simulink library "xps_library"  (R2018a)
settings: Solver=ode45  StartTime=0.0  StopTime=10.0  RelTol=1e-3
undefined symbols (not defined in the file or in its folder): ip_name, lib_path
libraries: xbsIndex_r4 x2548, casper_library_flow_control x68, simulink x52, $bdroot x22, casper_library_misc x9
(part 4 of 30)

== system xps_library/ADCs/adc_mkid_4x ==
  conv : Subsystem
      mask help:
      | Converts an (12-bit) unsigned number to 2's complement.
      | This block should eventually be able to handle arbitrary
      | width inputs.
  conv1 : Subsystem
      mask help:
      | Converts an (12-bit) unsigned number to 2's complement.
      | This block should eventually be able to handle arbitrary
      | width inputs.
  conv2 : Subsystem
      mask help:
      | Converts an (12-bit) unsigned number to 2's complement.
      | This block should eventually be able to handle arbitrary
      | width inputs.
  conv3 : Subsystem
      mask help:
      | Converts an (12-bit) unsigned number to 2's complement.
      | This block should eventually be able to handle arbitrary
      | width inputs.
  conv4 : Subsystem
      mask help:
      | Converts an (12-bit) unsigned number to 2's complement.
      | This block should eventually be able to handle arbitrary
      | width inputs.
  conv5 : Subsystem
      mask help:
      | Converts an (12-bit) unsigned number to 2's complement.
      | This block should eventually be able to handle arbitrary
      | width inputs.
  conv6 : Subsystem
      mask help:
      | Converts an (12-bit) unsigned number to 2's complement.
      | This block should eventually be able to handle arbitrary
      | width inputs.
  conv7 : Subsystem
      mask help:
      | Converts an (12-bit) unsigned number to 2's complement.
      | This block should eventually be able to handle arbitrary
      | width inputs.
  xps_library_ADCs_adc_mkid_4x_user_data_i{0..3} (4 alike) : xbsIndex_r4/Gateway In  gui_display_data_type=Fixed-point  arith_type=Unsigned  n_bits=12  bin_pt=0  preci_type=Single  exp_width=8  frac_width=24  rows=1  columns=1  quantization=Truncate  overflow=Wrap  period=1  UseAsADC=off  ADCChannel='1'  interface=None  automatic_assignment=on  address_offset=hex2dec('00')  intf_name=''  intf_description=''  default_value=0  timing_constraint=None  locs_specified=off  LOCs={}  io_standard={}  inherit_from_input=off  hdl_port=on  dbl_ovrd=off  block_type=gatewayin
      settings: infoedit="Gateway in block.  Converts inputs of type Simulink integer, double and fixed point to  Xilinx fixed point type.<P><P>Hardware notes:  In hardware these blocks become top level input ports."  xl_area=[0, 0, 0, 0, 0, 0, 0]  block_version=10.1.3
  xps_library_ADCs_adc_mkid_4x_user_data_q{0..3} (4 alike) : xbsIndex_r4/Gateway In  gui_display_data_type=Fixed-point  arith_type=Unsigned  n_bits=12  bin_pt=0  preci_type=Single  exp_width=8  frac_width=24  rows=1  columns=1  quantization=Truncate  overflow=Wrap  period=1  UseAsADC=off  ADCChannel='1'  interface=None  automatic_assignment=on  address_offset=hex2dec('00')  intf_name=''  intf_description=''  default_value=0  timing_constraint=None  locs_specified=off  LOCs={}  io_standard={}  inherit_from_input=off  hdl_port=on  dbl_ovrd=off  block_type=gatewayin
      settings: infoedit="Gateway in block.  Converts inputs of type Simulink integer, double and fixed point to  Xilinx fixed point type.<P><P>Hardware notes:  In hardware these blocks become top level input ports."  xl_area=[0, 0, 0, 0, 0, 0, 0]  block_version=10.1.3
  xps_library_ADCs_adc_mkid_4x_user_sync : xbsIndex_r4/Gateway In  gui_display_data_type=Fixed-point  arith_type=Boolean  n_bits=1  bin_pt=0  preci_type=Single  exp_width=8  frac_width=24  rows=1  columns=1  quantization=Truncate  overflow=Wrap  period=1  UseAsADC=off  ADCChannel='1'  interface=None  automatic_assignment=on  address_offset=hex2dec('00')  intf_name=''  intf_description=''  default_value=0  timing_constraint=None  locs_specified=off  LOCs={}  io_standard={}  inherit_from_input=off  hdl_port=on  dbl_ovrd=off  block_type=gatewayin
      settings: infoedit="Gateway in block.  Converts inputs of type Simulink integer, double and fixed point to  Xilinx fixed point type.<P><P>Hardware notes:  In hardware these blocks become top level input ports."  xl_area=[0, 0, 0, 0, 0, 0, 0]  block_version=10.1.3
  data_i0 : Outport
  data_i1 : Outport  Port=2
  data_i2 : Outport  Port=3
  data_i3 : Outport  Port=4
  data_q0 : Outport  Port=5
  data_q1 : Outport  Port=6
  data_q2 : Outport  Port=7
  data_q3 : Outport  Port=8
  sync : Outport  Port=9
  wires:
  xps_library_ADCs_adc_mkid_4x_user_data_q3/1 -> conv7/1(In1)
  conv7/1(Out1) -> data_q3/1
  xps_library_ADCs_adc_mkid_4x_user_data_q2/1 -> conv6/1(In1)
  conv6/1(Out1) -> data_q2/1
  xps_library_ADCs_adc_mkid_4x_user_data_i3/1 -> conv5/1(In1)
  conv5/1(Out1) -> data_i3/1
  xps_library_ADCs_adc_mkid_4x_user_data_i2/1 -> conv4/1(In1)
  conv4/1(Out1) -> data_i2/1
  xps_library_ADCs_adc_mkid_4x_user_sync/1 -> sync/1
  xps_library_ADCs_adc_mkid_4x_user_data_i0/1 -> conv/1(In1)
  conv/1(Out1) -> data_i0/1
  xps_library_ADCs_adc_mkid_4x_user_data_q0/1 -> conv2/1(In1)
  conv2/1(Out1) -> data_q0/1
  xps_library_ADCs_adc_mkid_4x_user_data_i1/1 -> conv1/1(In1)
  conv1/1(Out1) -> data_i1/1
  xps_library_ADCs_adc_mkid_4x_user_data_q1/1 -> conv3/1(In1)
  conv3/1(Out1) -> data_q1/1

== system xps_library/ADCs/adc_sim ==
  sim_adc_data_in : Inport
  adc_bias : Bias  Bias=128  SaturateOnIntegerOverflow=on
  adc_gain : Gain  Gain=128
  overflow_detector : $bdroot/ADCs/of_detect_bus  nStreams=8  bit_width=8
  sample0_ds : DownSample  N=8  phase=1
  sample1_ds : DownSample  N=8  phase=2
  sample2_ds : DownSample  N=8  phase=3
  sample3_ds : DownSample  N=8  phase=4
  sample4_ds : DownSample  N=8  phase=5
  sample5_ds : DownSample  N=8  phase=6
  sample6_ds : DownSample  N=8  phase=7
  sample7_ds : DownSample  N=8
  s0 : Outport
  s1 : Outport  Port=2
  s2 : Outport  Port=3
  s3 : Outport  Port=4
  s4 : Outport  Port=5
  s5 : Outport  Port=6
  s6 : Outport  Port=7
  s7 : Outport  Port=8
  of : Outport  Port=9
  wires:
  sim_adc_data_in/1 -> adc_gain/1
  adc_gain/1 -> adc_bias/1
  overflow_detector/1 -> of/1
  adc_bias/1 -> sample0_ds/1, sample1_ds/1, sample2_ds/1, sample3_ds/1, sample4_ds/1, sample5_ds/1, sample6_ds/1, sample7_ds/1
  sample0_ds/1 -> overflow_detector/1, s0/1
  sample1_ds/1 -> overflow_detector/2, s1/1
  sample2_ds/1 -> overflow_detector/3, s2/1
  sample3_ds/1 -> overflow_detector/4, s3/1
  sample4_ds/1 -> overflow_detector/5, s4/1
  sample5_ds/1 -> overflow_detector/6, s5/1
  sample6_ds/1 -> overflow_detector/7, s6/1
  sample7_ds/1 -> overflow_detector/8, s7/1

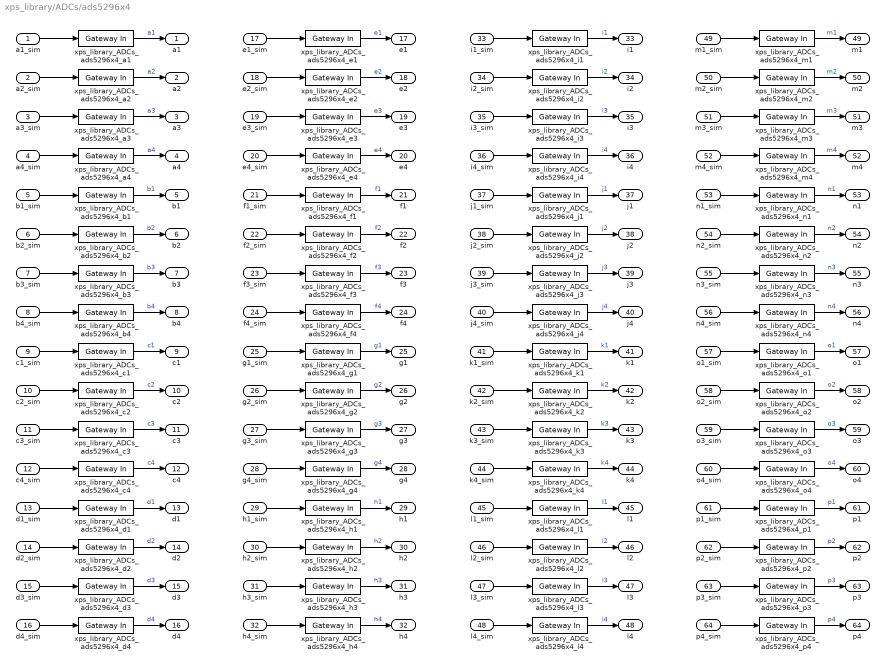
== system xps_library/ADCs/ads5296x4 ==
  a1_sim : Inport
  a2_sim : Inport  Port=2
  a3_sim : Inport  Port=3
  a4_sim : Inport  Port=4
  b1_sim : Inport  Port=5
  b2_sim : Inport  Port=6
  b3_sim : Inport  Port=7
  b4_sim : Inport  Port=8
  c1_sim : Inport  Port=9
  c2_sim : Inport  Port=10
  c3_sim : Inport  Port=11
  c4_sim : Inport  Port=12
  d1_sim : Inport  Port=13
  d2_sim : Inport  Port=14
  d3_sim : Inport  Port=15
  d4_sim : Inport  Port=16
  e1_sim : Inport  Port=17
  e2_sim : Inport  Port=18
  e3_sim : Inport  Port=19
  e4_sim : Inport  Port=20
  f1_sim : Inport  Port=21
  f2_sim : Inport  Port=22
  f3_sim : Inport  Port=23
  f4_sim : Inport  Port=24
  g1_sim : Inport  Port=25
  g2_sim : Inport  Port=26
  g3_sim : Inport  Port=27
  g4_sim : Inport  Port=28
  h1_sim : Inport  Port=29
  h2_sim : Inport  Port=30
  h3_sim : Inport  Port=31
  h4_sim : Inport  Port=32
  i1_sim : Inport  Port=33
  i2_sim : Inport  Port=34
  i3_sim : Inport  Port=35
  i4_sim : Inport  Port=36
  j1_sim : Inport  Port=37
  j2_sim : Inport  Port=38
  j3_sim : Inport  Port=39
  j4_sim : Inport  Port=40
  k1_sim : Inport  Port=41
  k2_sim : Inport  Port=42
  k3_sim : Inport  Port=43
  k4_sim : Inport  Port=44
  l1_sim : Inport  Port=45
  l2_sim : Inport  Port=46
  l3_sim : Inport  Port=47
  l4_sim : Inport  Port=48
  m1_sim : Inport  Port=49
  m2_sim : Inport  Port=50
  m3_sim : Inport  Port=51
  m4_sim : Inport  Port=52
  n1_sim : Inport  Port=53
  n2_sim : Inport  Port=54
  n3_sim : Inport  Port=55
  n4_sim : Inport  Port=56
  o1_sim : Inport  Port=57
  o2_sim : Inport  Port=58
  o3_sim : Inport  Port=59
  o4_sim : Inport  Port=60
  p1_sim : Inport  Port=61
  p2_sim : Inport  Port=62
  p3_sim : Inport  Port=63
  p4_sim : Inport  Port=64
  xps_library_ADCs_ads5296x4_a{1..4} (4 alike) : xbsIndex_r4/Gateway In  gui_display_data_type=Fixed-point  arith_type="Signed  (2's comp)"  n_bits=10  bin_pt=9  preci_type=Single  exp_width=8  frac_width=24  rows=1  columns=1  quantization="Round  (unbiased: +/- Inf)"  overflow=Saturate  period=1  UseAsADC=off  ADCChannel='1'  interface=None  automatic_assignment=on  address_offset=hex2dec('00')  intf_name=''  intf_description=''  default_value=0  timing_constraint=None  locs_specified=off  LOCs={}  io_standard={}  inherit_from_input=off  hdl_port=on  dbl_ovrd=off  block_type=gatewayin
  xps_library_ADCs_ads5296x4_b{1..4} (4 alike) : xbsIndex_r4/Gateway In  gui_display_data_type=Fixed-point  arith_type="Signed  (2's comp)"  n_bits=10  bin_pt=9  preci_type=Single  exp_width=8  frac_width=24  rows=1  columns=1  quantization="Round  (unbiased: +/- Inf)"  overflow=Saturate  period=1  UseAsADC=off  ADCChannel='1'  interface=None  automatic_assignment=on  address_offset=hex2dec('00')  intf_name=''  intf_description=''  default_value=0  timing_constraint=None  locs_specified=off  LOCs={}  io_standard={}  inherit_from_input=off  hdl_port=on  dbl_ovrd=off  block_type=gatewayin
  xps_library_ADCs_ads5296x4_c{1..4} (4 alike) : xbsIndex_r4/Gateway In  gui_display_data_type=Fixed-point  arith_type="Signed  (2's comp)"  n_bits=10  bin_pt=9  preci_type=Single  exp_width=8  frac_width=24  rows=1  columns=1  quantization="Round  (unbiased: +/- Inf)"  overflow=Saturate  period=1  UseAsADC=off  ADCChannel='1'  interface=None  automatic_assignment=on  address_offset=hex2dec('00')  intf_name=''  intf_description=''  default_value=0  timing_constraint=None  locs_specified=off  LOCs={}  io_standard={}  inherit_from_input=off  hdl_port=on  dbl_ovrd=off  block_type=gatewayin
  xps_library_ADCs_ads5296x4_d{1..4} (4 alike) : xbsIndex_r4/Gateway In  gui_display_data_type=Fixed-point  arith_type="Signed  (2's comp)"  n_bits=10  bin_pt=9  preci_type=Single  exp_width=8  frac_width=24  rows=1  columns=1  quantization="Round  (unbiased: +/- Inf)"  overflow=Saturate  period=1  UseAsADC=off  ADCChannel='1'  interface=None  automatic_assignment=on  address_offset=hex2dec('00')  intf_name=''  intf_description=''  default_value=0  timing_constraint=None  locs_specified=off  LOCs={}  io_standard={}  inherit_from_input=off  hdl_port=on  dbl_ovrd=off  block_type=gatewayin
  xps_library_ADCs_ads5296x4_e{1..4} (4 alike) : xbsIndex_r4/Gateway In  gui_display_data_type=Fixed-point  arith_type="Signed  (2's comp)"  n_bits=10  bin_pt=9  preci_type=Single  exp_width=8  frac_width=24  rows=1  columns=1  quantization="Round  (unbiased: +/- Inf)"  overflow=Saturate  period=1  UseAsADC=off  ADCChannel='1'  interface=None  automatic_assignment=on  address_offset=hex2dec('00')  intf_name=''  intf_description=''  default_value=0  timing_constraint=None  locs_specified=off  LOCs={}  io_standard={}  inherit_from_input=off  hdl_port=on  dbl_ovrd=off  block_type=gatewayin
  xps_library_ADCs_ads5296x4_f{1..4} (4 alike) : xbsIndex_r4/Gateway In  gui_display_data_type=Fixed-point  arith_type="Signed  (2's comp)"  n_bits=10  bin_pt=9  preci_type=Single  exp_width=8  frac_width=24  rows=1  columns=1  quantization="Round  (unbiased: +/- Inf)"  overflow=Saturate  period=1  UseAsADC=off  ADCChannel='1'  interface=None  automatic_assignment=on  address_offset=hex2dec('00')  intf_name=''  intf_description=''  default_value=0  timing_constraint=None  locs_specified=off  LOCs={}  io_standard={}  inherit_from_input=off  hdl_port=on  dbl_ovrd=off  block_type=gatewayin
  xps_library_ADCs_ads5296x4_g{1..4} (4 alike) : xbsIndex_r4/Gateway In  gui_display_data_type=Fixed-point  arith_type="Signed  (2's comp)"  n_bits=10  bin_pt=9  preci_type=Single  exp_width=8  frac_width=24  rows=1  columns=1  quantization="Round  (unbiased: +/- Inf)"  overflow=Saturate  period=1  UseAsADC=off  ADCChannel='1'  interface=None  automatic_assignment=on  address_offset=hex2dec('00')  intf_name=''  intf_description=''  default_value=0  timing_constraint=None  locs_specified=off  LOCs={}  io_standard={}  inherit_from_input=off  hdl_port=on  dbl_ovrd=off  block_type=gatewayin
  xps_library_ADCs_ads5296x4_h{1..4} (4 alike) : xbsIndex_r4/Gateway In  gui_display_data_type=Fixed-point  arith_type="Signed  (2's comp)"  n_bits=10  bin_pt=9  preci_type=Single  exp_width=8  frac_width=24  rows=1  columns=1  quantization="Round  (unbiased: +/- Inf)"  overflow=Saturate  period=1  UseAsADC=off  ADCChannel='1'  interface=None  automatic_assignment=on  address_offset=hex2dec('00')  intf_name=''  intf_description=''  default_value=0  timing_constraint=None  locs_specified=off  LOCs={}  io_standard={}  inherit_from_input=off  hdl_port=on  dbl_ovrd=off  block_type=gatewayin
  xps_library_ADCs_ads5296x4_i{1..4} (4 alike) : xbsIndex_r4/Gateway In  gui_display_data_type=Fixed-point  arith_type="Signed  (2's comp)"  n_bits=10  bin_pt=9  preci_type=Single  exp_width=8  frac_width=24  rows=1  columns=1  quantization="Round  (unbiased: +/- Inf)"  overflow=Saturate  period=1  UseAsADC=off  ADCChannel='1'  interface=None  automatic_assignment=on  address_offset=hex2dec('00')  intf_name=''  intf_description=''  default_value=0  timing_constraint=None  locs_specified=off  LOCs={}  io_standard={}  inherit_from_input=off  hdl_port=on  dbl_ovrd=off  block_type=gatewayin
  xps_library_ADCs_ads5296x4_j{1..4} (4 alike) : xbsIndex_r4/Gateway In  gui_display_data_type=Fixed-point  arith_type="Signed  (2's comp)"  n_bits=10  bin_pt=9  preci_type=Single  exp_width=8  frac_width=24  rows=1  columns=1  quantization="Round  (unbiased: +/- Inf)"  overflow=Saturate  period=1  UseAsADC=off  ADCChannel='1'  interface=None  automatic_assignment=on  address_offset=hex2dec('00')  intf_name=''  intf_description=''  default_value=0  timing_constraint=None  locs_specified=off  LOCs={}  io_standard={}  inherit_from_input=off  hdl_port=on  dbl_ovrd=off  block_type=gatewayin
  xps_library_ADCs_ads5296x4_k{1..4} (4 alike) : xbsIndex_r4/Gateway In  gui_display_data_type=Fixed-point  arith_type="Signed  (2's comp)"  n_bits=10  bin_pt=9  preci_type=Single  exp_width=8  frac_width=24  rows=1  columns=1  quantization="Round  (unbiased: +/- Inf)"  overflow=Saturate  period=1  UseAsADC=off  ADCChannel='1'  interface=None  automatic_assignment=on  address_offset=hex2dec('00')  intf_name=''  intf_description=''  default_value=0  timing_constraint=None  locs_specified=off  LOCs={}  io_standard={}  inherit_from_input=off  hdl_port=on  dbl_ovrd=off  block_type=gatewayin
  xps_library_ADCs_ads5296x4_l{1..4} (4 alike) : xbsIndex_r4/Gateway In  gui_display_data_type=Fixed-point  arith_type="Signed  (2's comp)"  n_bits=10  bin_pt=9  preci_type=Single  exp_width=8  frac_width=24  rows=1  columns=1  quantization="Round  (unbiased: +/- Inf)"  overflow=Saturate  period=1  UseAsADC=off  ADCChannel='1'  interface=None  automatic_assignment=on  address_offset=hex2dec('00')  intf_name=''  intf_description=''  default_value=0  timing_constraint=None  locs_specified=off  LOCs={}  io_standard={}  inherit_from_input=off  hdl_port=on  dbl_ovrd=off  block_type=gatewayin
  xps_library_ADCs_ads5296x4_m{1..4} (4 alike) : xbsIndex_r4/Gateway In  gui_display_data_type=Fixed-point  arith_type="Signed  (2's comp)"  n_bits=10  bin_pt=9  preci_type=Single  exp_width=8  frac_width=24  rows=1  columns=1  quantization="Round  (unbiased: +/- Inf)"  overflow=Saturate  period=1  UseAsADC=off  ADCChannel='1'  interface=None  automatic_assignment=on  address_offset=hex2dec('00')  intf_name=''  intf_description=''  default_value=0  timing_constraint=None  locs_specified=off  LOCs={}  io_standard={}  inherit_from_input=off  hdl_port=on  dbl_ovrd=off  block_type=gatewayin
  xps_library_ADCs_ads5296x4_n{1..4} (4 alike) : xbsIndex_r4/Gateway In  gui_display_data_type=Fixed-point  arith_type="Signed  (2's comp)"  n_bits=10  bin_pt=9  preci_type=Single  exp_width=8  frac_width=24  rows=1  columns=1  quantization="Round  (unbiased: +/- Inf)"  overflow=Saturate  period=1  UseAsADC=off  ADCChannel='1'  interface=None  automatic_assignment=on  address_offset=hex2dec('00')  intf_name=''  intf_description=''  default_value=0  timing_constraint=None  locs_specified=off  LOCs={}  io_standard={}  inherit_from_input=off  hdl_port=on  dbl_ovrd=off  block_type=gatewayin
  xps_library_ADCs_ads5296x4_o{1..4} (4 alike) : xbsIndex_r4/Gateway In  gui_display_data_type=Fixed-point  arith_type="Signed  (2's comp)"  n_bits=10  bin_pt=9  preci_type=Single  exp_width=8  frac_width=24  rows=1  columns=1  quantization="Round  (unbiased: +/- Inf)"  overflow=Saturate  period=1  UseAsADC=off  ADCChannel='1'  interface=None  automatic_assignment=on  address_offset=hex2dec('00')  intf_name=''  intf_description=''  default_value=0  timing_constraint=None  locs_specified=off  LOCs={}  io_standard={}  inherit_from_input=off  hdl_port=on  dbl_ovrd=off  block_type=gatewayin
  xps_library_ADCs_ads5296x4_p{1..4} (4 alike) : xbsIndex_r4/Gateway In  gui_display_data_type=Fixed-point  arith_type="Signed  (2's comp)"  n_bits=10  bin_pt=9  preci_type=Single  exp_width=8  frac_width=24  rows=1  columns=1  quantization="Round  (unbiased: +/- Inf)"  overflow=Saturate  period=1  UseAsADC=off  ADCChannel='1'  interface=None  automatic_assignment=on  address_offset=hex2dec('00')  intf_name=''  intf_description=''  default_value=0  timing_constraint=None  locs_specified=off  LOCs={}  io_standard={}  inherit_from_input=off  hdl_port=on  dbl_ovrd=off  block_type=gatewayin
  a1 : Outport
  a2 : Outport  Port=2
  a3 : Outport  Port=3
  a4 : Outport  Port=4
  b1 : Outport  Port=5
  b2 : Outport  Port=6
  b3 : Outport  Port=7
  b4 : Outport  Port=8
  c1 : Outport  Port=9
  c2 : Outport  Port=10
  c3 : Outport  Port=11
  c4 : Outport  Port=12
  d1 : Outport  Port=13
  d2 : Outport  Port=14
  d3 : Outport  Port=15
  d4 : Outport  Port=16
  e1 : Outport  Port=17
  e2 : Outport  Port=18
  e3 : Outport  Port=19
  e4 : Outport  Port=20
  f1 : Outport  Port=21
  f2 : Outport  Port=22
  f3 : Outport  Port=23
  f4 : Outport  Port=24
  g1 : Outport  Port=25
  g2 : Outport  Port=26
  g3 : Outport  Port=27
  g4 : Outport  Port=28
  h1 : Outport  Port=29
  h2 : Outport  Port=30
  h3 : Outport  Port=31
  h4 : Outport  Port=32
  i1 : Outport  Port=33
  i2 : Outport  Port=34
  i3 : Outport  Port=35
  i4 : Outport  Port=36
  j1 : Outport  Port=37
  j2 : Outport  Port=38
  j3 : Outport  Port=39
  j4 : Outport  Port=40
  k1 : Outport  Port=41
  k2 : Outport  Port=42
  k3 : Outport  Port=43
  k4 : Outport  Port=44
  l1 : Outport  Port=45
  l2 : Outport  Port=46
  l3 : Outport  Port=47
  l4 : Outport  Port=48
  m1 : Outport  Port=49
  m2 : Outport  Port=50
  m3 : Outport  Port=51
  m4 : Outport  Port=52
  n1 : Outport  Port=53
  n2 : Outport  Port=54
  n3 : Outport  Port=55
  n4 : Outport  Port=56
  o1 : Outport  Port=57
  o2 : Outport  Port=58
  o3 : Outport  Port=59
  o4 : Outport  Port=60
  p1 : Outport  Port=61
  p2 : Outport  Port=62
  p3 : Outport  Port=63
  p4 : Outport  Port=64
  wires:
  a1_sim/1 -> xps_library_ADCs_ads5296x4_a1/1
  xps_library_ADCs_ads5296x4_a1/1 -> a1/1  "a1"
  a2_sim/1 -> xps_library_ADCs_ads5296x4_a2/1
  xps_library_ADCs_ads5296x4_a2/1 -> a2/1  "a2"
  a3_sim/1 -> xps_library_ADCs_ads5296x4_a3/1
  xps_library_ADCs_ads5296x4_a3/1 -> a3/1  "a3"
  a4_sim/1 -> xps_library_ADCs_ads5296x4_a4/1
  xps_library_ADCs_ads5296x4_a4/1 -> a4/1  "a4"
  b1_sim/1 -> xps_library_ADCs_ads5296x4_b1/1
  xps_library_ADCs_ads5296x4_b1/1 -> b1/1  "b1"
  b2_sim/1 -> xps_library_ADCs_ads5296x4_b2/1
  xps_library_ADCs_ads5296x4_b2/1 -> b2/1  "b2"
  b3_sim/1 -> xps_library_ADCs_ads5296x4_b3/1
  xps_library_ADCs_ads5296x4_b3/1 -> b3/1  "b3"
  b4_sim/1 -> xps_library_ADCs_ads5296x4_b4/1
  xps_library_ADCs_ads5296x4_b4/1 -> b4/1  "b4"
  c1_sim/1 -> xps_library_ADCs_ads5296x4_c1/1
  xps_library_ADCs_ads5296x4_c1/1 -> c1/1  "c1"
  c2_sim/1 -> xps_library_ADCs_ads5296x4_c2/1
  xps_library_ADCs_ads5296x4_c2/1 -> c2/1  "c2"
  c3_sim/1 -> xps_library_ADCs_ads5296x4_c3/1
  xps_library_ADCs_ads5296x4_c3/1 -> c3/1  "c3"
  c4_sim/1 -> xps_library_ADCs_ads5296x4_c4/1
  xps_library_ADCs_ads5296x4_c4/1 -> c4/1  "c4"
  d1_sim/1 -> xps_library_ADCs_ads5296x4_d1/1
  xps_library_ADCs_ads5296x4_d1/1 -> d1/1  "d1"
  d2_sim/1 -> xps_library_ADCs_ads5296x4_d2/1
  xps_library_ADCs_ads5296x4_d2/1 -> d2/1  "d2"
  d3_sim/1 -> xps_library_ADCs_ads5296x4_d3/1
  xps_library_ADCs_ads5296x4_d3/1 -> d3/1  "d3"
  d4_sim/1 -> xps_library_ADCs_ads5296x4_d4/1
  xps_library_ADCs_ads5296x4_d4/1 -> d4/1  "d4"
  e1_sim/1 -> xps_library_ADCs_ads5296x4_e1/1
  xps_library_ADCs_ads5296x4_e1/1 -> e1/1  "e1"
  e2_sim/1 -> xps_library_ADCs_ads5296x4_e2/1
  xps_library_ADCs_ads5296x4_e2/1 -> e2/1  "e2"
  e3_sim/1 -> xps_library_ADCs_ads5296x4_e3/1
  xps_library_ADCs_ads5296x4_e3/1 -> e3/1  "e3"
  e4_sim/1 -> xps_library_ADCs_ads5296x4_e4/1
  xps_library_ADCs_ads5296x4_e4/1 -> e4/1  "e4"
  f1_sim/1 -> xps_library_ADCs_ads5296x4_f1/1
  xps_library_ADCs_ads5296x4_f1/1 -> f1/1  "f1"
  f2_sim/1 -> xps_library_ADCs_ads5296x4_f2/1
  xps_library_ADCs_ads5296x4_f2/1 -> f2/1  "f2"
  f3_sim/1 -> xps_library_ADCs_ads5296x4_f3/1
  xps_library_ADCs_ads5296x4_f3/1 -> f3/1  "f3"
  f4_sim/1 -> xps_library_ADCs_ads5296x4_f4/1
  xps_library_ADCs_ads5296x4_f4/1 -> f4/1  "f4"
  g1_sim/1 -> xps_library_ADCs_ads5296x4_g1/1
  xps_library_ADCs_ads5296x4_g1/1 -> g1/1  "g1"
  g2_sim/1 -> xps_library_ADCs_ads5296x4_g2/1
  xps_library_ADCs_ads5296x4_g2/1 -> g2/1  "g2"
  g3_sim/1 -> xps_library_ADCs_ads5296x4_g3/1
  xps_library_ADCs_ads5296x4_g3/1 -> g3/1  "g3"
  g4_sim/1 -> xps_library_ADCs_ads5296x4_g4/1
  xps_library_ADCs_ads5296x4_g4/1 -> g4/1  "g4"
  h1_sim/1 -> xps_library_ADCs_ads5296x4_h1/1
  xps_library_ADCs_ads5296x4_h1/1 -> h1/1  "h1"
  h2_sim/1 -> xps_library_ADCs_ads5296x4_h2/1
  xps_library_ADCs_ads5296x4_h2/1 -> h2/1  "h2"
  h3_sim/1 -> xps_library_ADCs_ads5296x4_h3/1
  xps_library_ADCs_ads5296x4_h3/1 -> h3/1  "h3"
  h4_sim/1 -> xps_library_ADCs_ads5296x4_h4/1
  xps_library_ADCs_ads5296x4_h4/1 -> h4/1  "h4"
  i1_sim/1 -> xps_library_ADCs_ads5296x4_i1/1
  xps_library_ADCs_ads5296x4_i1/1 -> i1/1  "i1"
  i2_sim/1 -> xps_library_ADCs_ads5296x4_i2/1
  xps_library_ADCs_ads5296x4_i2/1 -> i2/1  "i2"
  i3_sim/1 -> xps_library_ADCs_ads5296x4_i3/1
  xps_library_ADCs_ads5296x4_i3/1 -> i3/1  "i3"
  i4_sim/1 -> xps_library_ADCs_ads5296x4_i4/1
  xps_library_ADCs_ads5296x4_i4/1 -> i4/1  "i4"
  j1_sim/1 -> xps_library_ADCs_ads5296x4_j1/1
  xps_library_ADCs_ads5296x4_j1/1 -> j1/1  "j1"
  j2_sim/1 -> xps_library_ADCs_ads5296x4_j2/1
  xps_library_ADCs_ads5296x4_j2/1 -> j2/1  "j2"
  j3_sim/1 -> xps_library_ADCs_ads5296x4_j3/1
  xps_library_ADCs_ads5296x4_j3/1 -> j3/1  "j3"
  j4_sim/1 -> xps_library_ADCs_ads5296x4_j4/1
  xps_library_ADCs_ads5296x4_j4/1 -> j4/1  "j4"
  k1_sim/1 -> xps_library_ADCs_ads5296x4_k1/1
  xps_library_ADCs_ads5296x4_k1/1 -> k1/1  "k1"
  k2_sim/1 -> xps_library_ADCs_ads5296x4_k2/1
  xps_library_ADCs_ads5296x4_k2/1 -> k2/1  "k2"
  k3_sim/1 -> xps_library_ADCs_ads5296x4_k3/1
  xps_library_ADCs_ads5296x4_k3/1 -> k3/1  "k3"
  k4_sim/1 -> xps_library_ADCs_ads5296x4_k4/1
  xps_library_ADCs_ads5296x4_k4/1 -> k4/1  "k4"
  l1_sim/1 -> xps_library_ADCs_ads5296x4_l1/1
  xps_library_ADCs_ads5296x4_l1/1 -> l1/1  "l1"
  l2_sim/1 -> xps_library_ADCs_ads5296x4_l2/1
  xps_library_ADCs_ads5296x4_l2/1 -> l2/1  "l2"
  l3_sim/1 -> xps_library_ADCs_ads5296x4_l3/1
  xps_library_ADCs_ads5296x4_l3/1 -> l3/1  "l3"
  l4_sim/1 -> xps_library_ADCs_ads5296x4_l4/1
  xps_library_ADCs_ads5296x4_l4/1 -> l4/1  "l4"
  m1_sim/1 -> xps_library_ADCs_ads5296x4_m1/1
  xps_library_ADCs_ads5296x4_m1/1 -> m1/1  "m1"
  m2_sim/1 -> xps_library_ADCs_ads5296x4_m2/1
  xps_library_ADCs_ads5296x4_m2/1 -> m2/1  "m2"
  m3_sim/1 -> xps_library_ADCs_ads5296x4_m3/1
  xps_library_ADCs_ads5296x4_m3/1 -> m3/1  "m3"
  m4_sim/1 -> xps_library_ADCs_ads5296x4_m4/1
  xps_library_ADCs_ads5296x4_m4/1 -> m4/1  "m4"
  n1_sim/1 -> xps_library_ADCs_ads5296x4_n1/1
  xps_library_ADCs_ads5296x4_n1/1 -> n1/1  "n1"
  n2_sim/1 -> xps_library_ADCs_ads5296x4_n2/1
  xps_library_ADCs_ads5296x4_n2/1 -> n2/1  "n2"
  n3_sim/1 -> xps_library_ADCs_ads5296x4_n3/1
  xps_library_ADCs_ads5296x4_n3/1 -> n3/1  "n3"
  n4_sim/1 -> xps_library_ADCs_ads5296x4_n4/1
  xps_library_ADCs_ads5296x4_n4/1 -> n4/1  "n4"
  o1_sim/1 -> xps_library_ADCs_ads5296x4_o1/1
  xps_library_ADCs_ads5296x4_o1/1 -> o1/1  "o1"
  o2_sim/1 -> xps_library_ADCs_ads5296x4_o2/1
  xps_library_ADCs_ads5296x4_o2/1 -> o2/1  "o2"
  o3_sim/1 -> xps_library_ADCs_ads5296x4_o3/1
  xps_library_ADCs_ads5296x4_o3/1 -> o3/1  "o3"
  o4_sim/1 -> xps_library_ADCs_ads5296x4_o4/1
  xps_library_ADCs_ads5296x4_o4/1 -> o4/1  "o4"
  p1_sim/1 -> xps_library_ADCs_ads5296x4_p1/1
  xps_library_ADCs_ads5296x4_p1/1 -> p1/1  "p1"
  p2_sim/1 -> xps_library_ADCs_ads5296x4_p2/1
  xps_library_ADCs_ads5296x4_p2/1 -> p2/1  "p2"
  p3_sim/1 -> xps_library_ADCs_ads5296x4_p3/1
  xps_library_ADCs_ads5296x4_p3/1 -> p3/1  "p3"
  p4_sim/1 -> xps_library_ADCs_ads5296x4_p4/1
  xps_library_ADCs_ads5296x4_p4/1 -> p4/1  "p4"

== system xps_library/ADCs/asiaa_adc5g ==
  sim_a : Inport
  sim_sync : Inport  Port=2
  bias_a : Bias  Bias=8  SaturateOnIntegerOverflow=on
  delay_a0 : Delay  InitialCondition=0  InputProcessing=Inherited
  delay_a{1..15} (15 alike) : Delay  DelayLength=1  InitialCondition=0  InputProcessing=Inherited
  downsample_a0 : DownSample  N=16  RateOptions=Allow multirate processing
  downsample_a1 : DownSample  N=16  phase=1  RateOptions=Allow multirate processing
  downsample_a10 : DownSample  N=16  phase=10  RateOptions=Allow multirate processing
  downsample_a11 : DownSample  N=16  phase=11  RateOptions=Allow multirate processing
  downsample_a12 : DownSample  N=16  phase=12  RateOptions=Allow multirate processing
  downsample_a13 : DownSample  N=16  phase=13  RateOptions=Allow multirate processing
  downsample_a14 : DownSample  N=16  phase=14  RateOptions=Allow multirate processing
  downsample_a15 : DownSample  N=16  phase=15  RateOptions=Allow multirate processing
  downsample_a2 : DownSample  N=16  phase=2  RateOptions=Allow multirate processing
  downsample_a3 : DownSample  N=16  phase=3  RateOptions=Allow multirate processing
  downsample_a4 : DownSample  N=16  phase=4  RateOptions=Allow multirate processing
  downsample_a5 : DownSample  N=16  phase=5  RateOptions=Allow multirate processing
  downsample_a6 : DownSample  N=16  phase=6  RateOptions=Allow multirate processing
  downsample_a7 : DownSample  N=16  phase=7  RateOptions=Allow multirate processing
  downsample_a8 : DownSample  N=16  phase=8  RateOptions=Allow multirate processing
  downsample_a9 : DownSample  N=16  phase=9  RateOptions=Allow multirate processing
  gain_a : Gain  Gain=8  SaturateOnIntegerOverflow=on  OutDataTypeStr=Inherit: Same as input  ParamDataTypeStr=Inherit: Same as input
  xps_library_ADCs_asiaa_adc5g_sync : xbsIndex_r4/Gateway In  gui_display_data_type=Fixed-point  arith_type=Boolean  n_bits=16  bin_pt=14  preci_type=Single  exp_width=8  frac_width=24  rows=1  columns=1  quantization="Round  (unbiased: +/- Inf)"  overflow=Saturate  period=1  UseAsADC=off  ADCChannel='1'  interface=None  automatic_assignment=on  address_offset=hex2dec('00')  intf_name=''  intf_description=''  default_value=0  timing_constraint=None  locs_specified=off  LOCs={}  io_standard={}  inherit_from_input=off  hdl_port=on  dbl_ovrd=off  block_type=gatewayin
  xps_library_ADCs_asiaa_adc5g_user_data_i{0..7} (8 alike) : xbsIndex_r4/Gateway In  gui_display_data_type=Fixed-point  arith_type=Unsigned  n_bits=4  bin_pt=0  preci_type=Single  exp_width=8  frac_width=24  rows=1  columns=1  quantization=Truncate  overflow=Wrap  period=1  UseAsADC=off  ADCChannel='1'  interface=None  automatic_assignment=on  address_offset=hex2dec('00')  intf_name=''  intf_description=''  default_value=0  timing_constraint=None  locs_specified=off  LOCs={}  io_standard={}  inherit_from_input=off  hdl_port=on  dbl_ovrd=off  block_type=gatewayin
  xps_library_ADCs_asiaa_adc5g_user_data_q{0..7} (8 alike) : xbsIndex_r4/Gateway In  gui_display_data_type=Fixed-point  arith_type=Unsigned  n_bits=4  bin_pt=0  preci_type=Single  exp_width=8  frac_width=24  rows=1  columns=1  quantization=Truncate  overflow=Wrap  period=1  UseAsADC=off  ADCChannel='1'  interface=None  automatic_assignment=on  address_offset=hex2dec('00')  intf_name=''  intf_description=''  default_value=0  timing_constraint=None  locs_specified=off  LOCs={}  io_standard={}  inherit_from_input=off  hdl_port=on  dbl_ovrd=off  block_type=gatewayin
  a0 : Outport
  a1 : Outport  Port=2
  a2 : Outport  Port=3
  a3 : Outport  Port=4
  a4 : Outport  Port=5
  a5 : Outport  Port=6
  a6 : Outport  Port=7
  a7 : Outport  Port=8
  a8 : Outport  Port=9
  a9 : Outport  Port=10
  a10 : Outport  Port=11
  a11 : Outport  Port=12
  a12 : Outport  Port=13
  a13 : Outport  Port=14
  a14 : Outport  Port=15
  a15 : Outport  Port=16
  sync_out : Outport  Port=17
  wires:
  sim_a/1 -> gain_a/1
  gain_a/1 -> bias_a/1
  bias_a/1 -> downsample_a0/1, downsample_a1/1, downsample_a2/1, downsample_a3/1, downsample_a4/1, downsample_a5/1, downsample_a6/1, downsample_a7/1, downsample_a8/1, downsample_a9/1, downsample_a10/1, downsample_a11/1, downsample_a12/1, downsample_a13/1, downsample_a14/1, downsample_a15/1
  downsample_a0/1 -> delay_a0/1
  delay_a0/1 -> xps_library_ADCs_asiaa_adc5g_user_data_i0/1
  xps_library_ADCs_asiaa_adc5g_user_data_i0/1 -> a0/1
  downsample_a1/1 -> delay_a1/1
  delay_a1/1 -> xps_library_ADCs_asiaa_adc5g_user_data_i1/1
  xps_library_ADCs_asiaa_adc5g_user_data_i1/1 -> a1/1
  downsample_a2/1 -> delay_a2/1
  delay_a2/1 -> xps_library_ADCs_asiaa_adc5g_user_data_i2/1
  xps_library_ADCs_asiaa_adc5g_user_data_i2/1 -> a2/1
  downsample_a3/1 -> delay_a3/1
  delay_a3/1 -> xps_library_ADCs_asiaa_adc5g_user_data_i3/1
  xps_library_ADCs_asiaa_adc5g_user_data_i3/1 -> a3/1
  downsample_a4/1 -> delay_a4/1
  delay_a4/1 -> xps_library_ADCs_asiaa_adc5g_user_data_i4/1
  xps_library_ADCs_asiaa_adc5g_user_data_i4/1 -> a4/1
  downsample_a5/1 -> delay_a5/1
  delay_a5/1 -> xps_library_ADCs_asiaa_adc5g_user_data_i5/1
  xps_library_ADCs_asiaa_adc5g_user_data_i5/1 -> a5/1
  downsample_a6/1 -> delay_a6/1
  delay_a6/1 -> xps_library_ADCs_asiaa_adc5g_user_data_i6/1
  xps_library_ADCs_asiaa_adc5g_user_data_i6/1 -> a6/1
  downsample_a7/1 -> delay_a7/1
  delay_a7/1 -> xps_library_ADCs_asiaa_adc5g_user_data_i7/1
  xps_library_ADCs_asiaa_adc5g_user_data_i7/1 -> a7/1
  downsample_a8/1 -> delay_a8/1
  delay_a8/1 -> xps_library_ADCs_asiaa_adc5g_user_data_q0/1
  xps_library_ADCs_asiaa_adc5g_user_data_q0/1 -> a8/1
  downsample_a9/1 -> delay_a9/1
  delay_a9/1 -> xps_library_ADCs_asiaa_adc5g_user_data_q1/1
  xps_library_ADCs_asiaa_adc5g_user_data_q1/1 -> a9/1
  downsample_a10/1 -> delay_a10/1
  delay_a10/1 -> xps_library_ADCs_asiaa_adc5g_user_data_q2/1
  xps_library_ADCs_asiaa_adc5g_user_data_q2/1 -> a10/1
  downsample_a11/1 -> delay_a11/1
  delay_a11/1 -> xps_library_ADCs_asiaa_adc5g_user_data_q3/1
  xps_library_ADCs_asiaa_adc5g_user_data_q3/1 -> a11/1
  downsample_a12/1 -> delay_a12/1
  delay_a12/1 -> xps_library_ADCs_asiaa_adc5g_user_data_q4/1
  xps_library_ADCs_asiaa_adc5g_user_data_q4/1 -> a12/1
  downsample_a13/1 -> delay_a13/1
  delay_a13/1 -> xps_library_ADCs_asiaa_adc5g_user_data_q5/1
  xps_library_ADCs_asiaa_adc5g_user_data_q5/1 -> a13/1
  downsample_a14/1 -> delay_a14/1
  delay_a14/1 -> xps_library_ADCs_asiaa_adc5g_user_data_q6/1
  xps_library_ADCs_asiaa_adc5g_user_data_q6/1 -> a14/1
  downsample_a15/1 -> delay_a15/1
  delay_a15/1 -> xps_library_ADCs_asiaa_adc5g_user_data_q7/1
  xps_library_ADCs_asiaa_adc5g_user_data_q7/1 -> a15/1
  sim_sync/1 -> xps_library_ADCs_asiaa_adc5g_sync/1
  xps_library_ADCs_asiaa_adc5g_sync/1 -> sync_out/1

== system xps_library/ADCs/conv ==
  In1 : Inport
  Concat : xbsIndex_r4/Concat  num_inputs=2  dbl_ovrd=off  block_type=concat
      settings: block_version=8.2.02
  Inverter : xbsIndex_r4/Inverter  en=off  latency=0  dbl_ovrd=off  block_type=inv
      settings: xl_area=[0, 0, 0, 0, 0, 0, 0]  block_version=8.2.02
  Reinterpret : xbsIndex_r4/Reinterpret  force_arith_type=on  arith_type="Signed  (2's comp)"  force_bin_pt=on  bin_pt=bit_width-1  block_type=reinterpret
      settings: infoedit="Changes signal type without altering the binary representation.   You can changed the signal between signed and unsigned, and relocate the binary point.<br><br>Hardware notes: In hardware this block costs nothing.<br><br>Example:  Suppose the input is 6 bits wide, signed, with 2 fractional bits, and the output is forced to unsigned with 0 fractional bits.  Then an input of -2.0 (1110.00 in binary 2's complement) becomes an output of 56 (111000 in binary)."  block_version=8.2.02
  Slice : xbsIndex_r4/Slice  nbits=1  boolean_output=off  mode=Upper Bit Location + Width  bit1=0  base1=MSB of Input  bit0=0  base0=LSB of Input  dbl_ovrd=off  block_type=slice
      settings: infoedit="Extracts a given range of bits from each input sample and presents it at the output.  The output type is ordinarily unsigned with binary point at zero, but can be Boolean when the slice is one bit wide.<P><P>Hardware notes: In hardware this block costs nothing."  block_version=8.2.02
  Slice1 : xbsIndex_r4/Slice  nbits=bit_width-1  boolean_output=off  mode=Lower Bit Location + Width  bit1=0  base1=MSB of Input  bit0=0  base0=LSB of Input  dbl_ovrd=off  block_type=slice
      settings: block_version=8.2.02
  Out1 : Outport
  wires:
  Reinterpret/1 -> Out1/1
  Concat/1 -> Reinterpret/1
  Slice1/1 -> Concat/2
  Inverter/1 -> Concat/1
  Slice/1 -> Inverter/1
  In1/1 -> Slice/1, Slice1/1

== system xps_library/ADCs/generic_adc ==
  sim_data0 : Inport
  sim_sync : Inport  Port=2
  bias0 : Bias  Bias=127.5  SaturateOnIntegerOverflow=on
  concat0_{0..3} (4 alike) : xbsIndex_r4/Concat  num_inputs=2  dbl_ovrd=off  block_type=concat
  d0_del0 : Delay  InputProcessing=Inherited
  d0_del1 : Delay  DelayLength=1  InputProcessing=Inherited
  d0_del2 : Delay  DelayLength=1  InputProcessing=Inherited
  d0_del3 : Delay  DelayLength=1  InputProcessing=Inherited
  d0_ds0 : DownSample  N=4  RateOptions=Allow multirate processing
  d0_ds1 : DownSample  N=4  phase=1  RateOptions=Allow multirate processing
  d0_ds2 : DownSample  N=4  phase=2  RateOptions=Allow multirate processing
  d0_ds3 : DownSample  N=4  phase=3  RateOptions=Allow multirate processing
  gain0 : Gain  Gain=127.5  SaturateOnIntegerOverflow=on  OutDataTypeStr=Inherit: Same as input  ParamDataTypeStr=Inherit: Same as input
  inv0_{0..3} (4 alike) : xbsIndex_r4/Inverter  en=off  latency=0  dbl_ovrd=off  block_type=inv
      settings: block_version=11.4
  reinterpret0_{0..3} (4 alike) : xbsIndex_r4/Reinterpret  force_arith_type=on  arith_type="Signed  (2's comp)"  force_bin_pt=on  bin_pt=7  block_type=reinterpret
      settings: infoedit="Changes signal type without altering the binary representation.   You can changed the signal between signed and unsigned, and relocate the binary point.<br><br>Hardware notes: In hardware this block costs nothing.<br><br>Example:  Suppose the input is 6 bits wide, signed, with 2 fractional bits, and the output is forced to unsigned with 0 fractional bits.  Then an input of -2.0 (1110.00 in binary 2's complement) becomes an output of 56 (111000 in binary)."
  sign0_{0..3} (4 alike) : xbsIndex_r4/Slice  nbits=1  boolean_output=off  mode=Upper Bit Location + Width  bit1=0  base1=MSB of Input  bit0=0  base0=MSB of Input  dbl_ovrd=off  block_type=slice
  sync_del0 : Delay  InputProcessing=Inherited
  sync_del1 : Delay  DelayLength=1  InputProcessing=Inherited
  sync_del2 : Delay  DelayLength=1  InputProcessing=Inherited
  sync_del3 : Delay  DelayLength=1  InputProcessing=Inherited
  sync_ds0 : DownSample  N=4  RateOptions=Allow multirate processing
  sync_ds1 : DownSample  N=4  phase=1  RateOptions=Allow multirate processing
  sync_ds2 : DownSample  N=4  phase=2  RateOptions=Allow multirate processing
  sync_ds3 : DownSample  N=4  phase=3  RateOptions=Allow multirate processing
  val0_{0..3} (4 alike) : xbsIndex_r4/Slice  nbits=7  boolean_output=off  mode=Lower Bit Location + Width  bit1=0  base1=LSB of Input  bit0=0  base0=LSB of Input  dbl_ovrd=off  block_type=slice
  xps_library_ADCs_generic_adc_user_data{0..3} (4 alike) : xbsIndex_r4/Gateway In  gui_display_data_type=Fixed-point  arith_type=Unsigned  n_bits=8  bin_pt=0  preci_type=Single  exp_width=8  frac_width=24  rows=1  columns=1  quantization="Round  (unbiased: +/- Inf)"  overflow=Saturate  period=1  UseAsADC=off  ADCChannel='1'  interface=None  automatic_assignment=on  address_offset=hex2dec('00')  intf_name=''  intf_description=''  default_value=0  timing_constraint=None  locs_specified=off  LOCs={}  io_standard={}  inherit_from_input=off  hdl_port=on  dbl_ovrd=off  block_type=gatewayin
  xps_library_ADCs_generic_adc_user_sync{0..3} (4 alike) : xbsIndex_r4/Gateway In  gui_display_data_type=Fixed-point  arith_type=Boolean  n_bits=16  bin_pt=14  preci_type=Single  exp_width=8  frac_width=24  rows=1  columns=1  quantization="Round  (unbiased: +/- Inf)"  overflow=Saturate  period=1  UseAsADC=off  ADCChannel='1'  interface=None  automatic_assignment=on  address_offset=hex2dec('00')  intf_name=''  intf_description=''  default_value=0  timing_constraint=None  locs_specified=off  LOCs={}  io_standard={}  inherit_from_input=off  hdl_port=on  dbl_ovrd=off  block_type=gatewayin
  data0_0 : Outport
  data0_1 : Outport  Port=2
  data0_2 : Outport  Port=3
  data0_3 : Outport  Port=4
  sync0 : Outport  Port=5
  sync1 : Outport  Port=6
  sync2 : Outport  Port=7
  sync3 : Outport  Port=8
  wires:
  sim_data0/1 -> gain0/1
  gain0/1 -> bias0/1
  bias0/1 -> d0_ds0/1, d0_ds1/1, d0_ds2/1, d0_ds3/1
  d0_ds0/1 -> d0_del0/1
  d0_del0/1 -> xps_library_ADCs_generic_adc_user_data0/1
  xps_library_ADCs_generic_adc_user_data0/1 -> sign0_0/1, val0_0/1
  sign0_0/1 -> inv0_0/1
  inv0_0/1 -> concat0_0/1
  val0_0/1 -> concat0_0/2
  concat0_0/1 -> reinterpret0_0/1
  reinterpret0_0/1 -> data0_0/1
  d0_ds1/1 -> d0_del1/1
  d0_del1/1 -> xps_library_ADCs_generic_adc_user_data1/1
  xps_library_ADCs_generic_adc_user_data1/1 -> sign0_1/1, val0_1/1
  sign0_1/1 -> inv0_1/1
  inv0_1/1 -> concat0_1/1
  val0_1/1 -> concat0_1/2
  concat0_1/1 -> reinterpret0_1/1
  reinterpret0_1/1 -> data0_1/1
  d0_ds2/1 -> d0_del2/1
  d0_del2/1 -> xps_library_ADCs_generic_adc_user_data2/1
  xps_library_ADCs_generic_adc_user_data2/1 -> sign0_2/1, val0_2/1
  sign0_2/1 -> inv0_2/1
  inv0_2/1 -> concat0_2/1
  val0_2/1 -> concat0_2/2
  concat0_2/1 -> reinterpret0_2/1
  reinterpret0_2/1 -> data0_2/1
  d0_ds3/1 -> d0_del3/1
  d0_del3/1 -> xps_library_ADCs_generic_adc_user_data3/1
  xps_library_ADCs_generic_adc_user_data3/1 -> sign0_3/1, val0_3/1
  sign0_3/1 -> inv0_3/1
  inv0_3/1 -> concat0_3/1
  val0_3/1 -> concat0_3/2
  concat0_3/1 -> reinterpret0_3/1
  reinterpret0_3/1 -> data0_3/1
  sim_sync/1 -> sync_ds0/1, sync_ds1/1, sync_ds2/1, sync_ds3/1
  sync_ds0/1 -> sync_del0/1
  sync_del0/1 -> xps_library_ADCs_generic_adc_user_sync0/1
  xps_library_ADCs_generic_adc_user_sync0/1 -> sync0/1
  sync_ds1/1 -> sync_del1/1
  sync_del1/1 -> xps_library_ADCs_generic_adc_user_sync1/1
  xps_library_ADCs_generic_adc_user_sync1/1 -> sync1/1
  sync_ds2/1 -> sync_del2/1
  sync_del2/1 -> xps_library_ADCs_generic_adc_user_sync2/1
  xps_library_ADCs_generic_adc_user_sync2/1 -> sync2/1
  sync_ds3/1 -> sync_del3/1
  sync_del3/1 -> xps_library_ADCs_generic_adc_user_sync3/1
  xps_library_ADCs_generic_adc_user_sync3/1 -> sync3/1
